simulink model "FullTrackTableModel"  (R2020b)
settings: Solver=VariableStepAuto  StartTime=0.0  StopTime=10.0  MaxStep=10E-2  RelTol=1e-3
settings Model: Creator=Authorized User  LastModifiedBy=joems

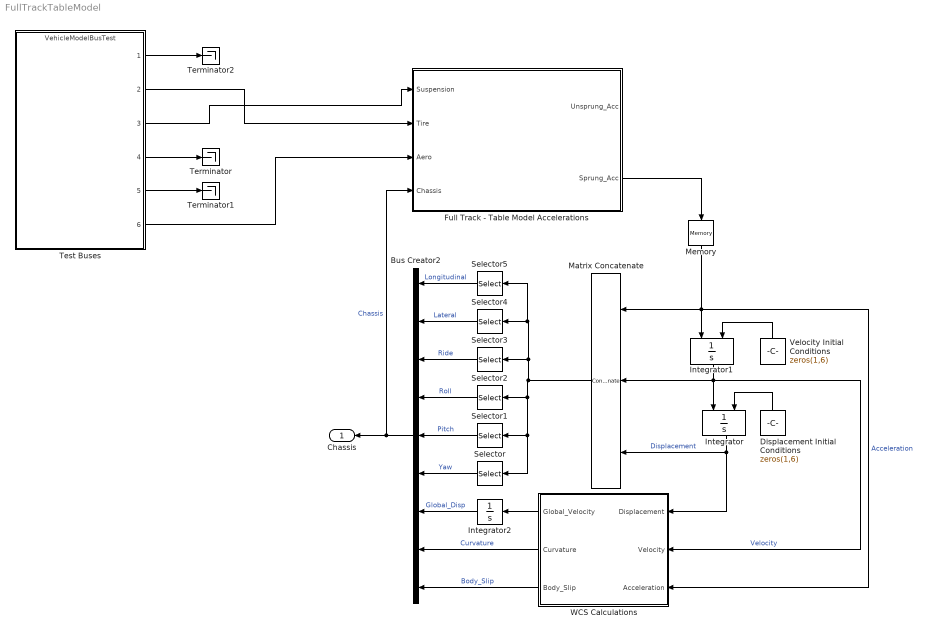
== system FullTrackTableModel ==
  Bus Creator2 : BusCreator  Inputs=9
  Displacement Initial Conditions : Constant  Value=zeros(1,6)
  Full Track - Table Model Accelerations : MATLAB Function  TreatAsAtomicUnit=on
  Integrator : Integrator  InitialConditionSource=external
  Integrator1 : Integrator  InitialConditionSource=external
  Integrator2 : Integrator
  Matrix Concatenate : Concatenate  NumInputs=3  Mode=Multidimensional array  ConcatenateDimension=2
  Memory : Memory
  Selector : Selector  NumberOfDimensions=2  InputPortWidth=3  IndexOptions=Index vector (dialog),Index vector (dialog)  Indices=6,[3 2 1]  OutputSizes=1,1
  Selector1 : Selector  NumberOfDimensions=2  InputPortWidth=3  IndexOptions=Index vector (dialog),Index vector (dialog)  Indices=5,[3 2 1]  OutputSizes=1,1
  Selector2 : Selector  NumberOfDimensions=2  InputPortWidth=3  IndexOptions=Index vector (dialog),Index vector (dialog)  Indices=4,[3 2 1]  OutputSizes=1,1
  Selector3 : Selector  NumberOfDimensions=2  InputPortWidth=3  IndexOptions=Index vector (dialog),Index vector (dialog)  Indices=3,[3 2 1]  OutputSizes=1,1
  Selector4 : Selector  NumberOfDimensions=2  InputPortWidth=3  IndexOptions=Index vector (dialog),Index vector (dialog)  Indices=2,[3 2 1]  OutputSizes=1,1
  Selector5 : Selector  NumberOfDimensions=2  InputPortWidth=3  IndexOptions=Index vector (dialog),Index vector (dialog)  Indices=1,[3 2 1]  OutputSizes=1,1
  Terminator : Terminator
  Terminator1 : Terminator
  Terminator2 : Terminator
  Test Buses : ModelReference  ModelNameDialog=VehicleModelBusTest.slx  SimulationMode=Normal  ModelReferenceVersion=1.30
  Velocity Initial Conditions : Constant  Value=zeros(1,6)
  WCS Calculations : MATLAB Function  TreatAsAtomicUnit=on
  Chassis : Outport  OutDataTypeStr=Bus: Chassis
  wires:
  Test Buses/6 -> Full Track - Table Model Accelerations/3(Aero)
  Test Buses/3 -> Full Track - Table Model Accelerations/1(Suspension)
  Test Buses/2 -> Full Track - Table Model Accelerations/2(Tire)
  Test Buses/4 -> Terminator/1
  Test Buses/5 -> Terminator1/1
  Bus Creator2/1 -> Chassis/1, Full Track - Table Model Accelerations/4(Chassis)  "Chassis"
  Matrix Concatenate/1 -> Selector5/1, Selector4/1, Selector3/1, Selector/1, Selector1/1, Selector2/1
  Integrator1/1 -> Integrator/1, WCS Calculations/2(Velocity), Matrix Concatenate/2  "Velocity"
  Integrator/1 -> WCS Calculations/1(Displacement), Matrix Concatenate/3  "Displacement"
  WCS Calculations/2(Curvature) -> Bus Creator2/8  "Curvature"
  WCS Calculations/3(Body_Slip) -> Bus Creator2/9  "Body_Slip"
  WCS Calculations/1(Global_Velocity) -> Integrator2/1
  Selector/1 -> Bus Creator2/6  "Yaw"
  Selector1/1 -> Bus Creator2/5  "Pitch"
  Selector2/1 -> Bus Creator2/4  "Roll"
  Selector3/1 -> Bus Creator2/3  "Ride"
  Selector4/1 -> Bus Creator2/2  "Lateral"
  Selector5/1 -> Bus Creator2/1  "Longitudinal"
  Test Buses/1 -> Terminator2/1
  Velocity Initial Conditions/1 -> Integrator1/2
  Displacement Initial Conditions/1 -> Integrator/2
  Integrator2/1 -> Bus Creator2/7  "Global_Disp"
  Memory/1 -> Integrator1/1, WCS Calculations/3(Acceleration), Matrix Concatenate/1  "Acceleration"
  Full Track - Table Model Accelerations/2(Sprung_Acc) -> Memory/1

== matlab function FullTrackTableModel/WCS Calculations ==
  data: Displacement input; Velocity input; Global_Velocity output; Curvature output; Body_Slip output; Acceleration input
function [Global_Velocity, Curvature, Body_Slip] = ...
    WCS_Calculations( Displacement, Velocity, Acceleration )
%% Nomenclature
% Yaw Angle                : Displacement(6)
% Longitudinal Velocity    : Velocity(1) 
% Longitudinal Acceleration: Acceleration(1)
% Lateral Velocity         : Velocity(2) 
% Lateral Acceleration     : Acceleration(2)

%% Global Displacement
Global_Velocity = zeros(1,2);

Global_Velocity(1) = Velocity(1) .* cosd( Displacement(6) ) - ...
                     Velocity(2) .* sind( Displacement(6) );
                 
Global_Velocity(2) = Velocity(1) .* sind( Displacement(6) ) + ...
                     Velocity(2) .* cosd( Displacement(6) );  
                 
%% Curvature
if abs(Velocity(1).^2 + Velocity(2).^2) <= 0.01;
    Curvature = 1000;
else
    Curvature = abs( Acceleration(1).*Velocity(2) - Velocity(1).*Acceleration(2) ) ./ ...
        ( Velocity(2).^2 + Velocity(2).^2 ).^(3/2);
end

%% Body Slip
Body_Slip = atan2d( Velocity(2), Velocity(1) );

end

== matlab function FullTrackTableModel/Full Track - Table Model Accelerations ==
  data: Suspension input; Tire input; Aero input; Chassis input; Unsprung_Acc output; Sprung_Acc output
function [Unsprung_Acc, Sprung_Acc] = ...
    Acceleration_Evaluation( Suspension, Tire, Aero, Chassis )
%% Initialization
Unsprung_Acc = zeros(4,1);
Sprung_Acc = zeros(6,1);

%% Longitudinal Dynamics
Sprung_Acc(1) = 1;

%% Lateral Dynamics
Sprung_Acc(2) = 1;

%% Ride Dynamics
Sprung_Acc(3) = 1;

%% Roll Dynamics
Sprung_Acc(4) = 0;

%% Pitch Dynamics
Sprung_Acc(5) = 1;

%% Yaw Dynamics
Sprung_Acc(6) = 1;
